simulink model "left_leg"  (R2014b)
settings: Solver=ode45  StartTime=0.0  StopTime=10  FixedStep=1e-4  RelTol=1e-3
undefined symbols (not defined in the file or in its folder): MX28_inertia, MX28_Te, X, Y, Z
libraries: sm_lib x39, nesl_utility x20
(part 1 of 2)
settings Model: Creator=florent  LastModifiedBy=florent
settings DebuggingCC: IntegerOverflowMsg=none  ParameterDowncastMsg=warning  ParameterPrecisionLossMsg=none  ParameterTunabilityLossMsg=none  StateNameClashWarn=warning  IntegerSaturationMsg=none

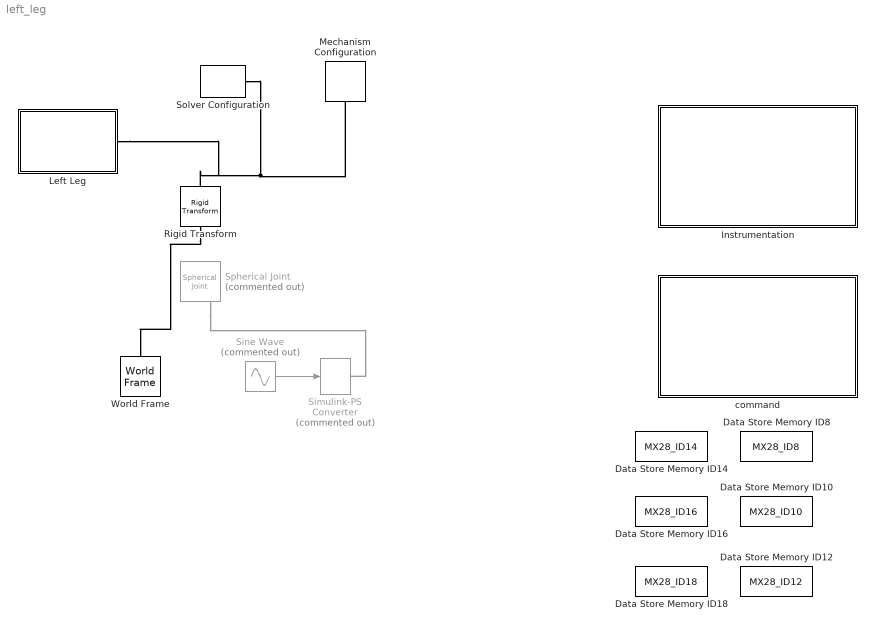
== system left_leg ==
  Data Store Memory ID10 : DataStoreMemory  DataStoreName=MX28_ID10  WriteAfterWriteMsg=error  InitialValue=MX28_default  VectorParams1D=off  OutDataTypeStr=Bus: MX28_bus
  Data Store Memory ID12 : DataStoreMemory  DataStoreName=MX28_ID12  WriteAfterWriteMsg=error  InitialValue=MX28_default  VectorParams1D=off  OutDataTypeStr=Bus: MX28_bus
  Data Store Memory ID14 : DataStoreMemory  DataStoreName=MX28_ID14  WriteAfterWriteMsg=error  InitialValue=MX28_default  VectorParams1D=off  OutDataTypeStr=Bus: MX28_bus
  Data Store Memory ID16 : DataStoreMemory  DataStoreName=MX28_ID16  WriteAfterWriteMsg=error  InitialValue=MX28_default  VectorParams1D=off  OutDataTypeStr=Bus: MX28_bus
  Data Store Memory ID18 : DataStoreMemory  DataStoreName=MX28_ID18  WriteAfterWriteMsg=error  InitialValue=MX28_default  VectorParams1D=off  OutDataTypeStr=Bus: MX28_bus
  Data Store Memory ID8 : DataStoreMemory  DataStoreName=MX28_ID8  WriteAfterWriteMsg=error  InitialValue=MX28_default  VectorParams1D=off  OutDataTypeStr=Bus: MX28_bus
  Instrumentation : Subsystem
  Left Leg : Subsystem
      mask init:
      | [ModelDir,~,~] = fileparts(which(gcs));
      | 
      | Block = [gcb '/Left Hip Yaw/Solid'];
      | STLFileName = [ModelDir filesep 'STL' filesep 'Hip1.STL'];
      | if ~strcmp(get_param(Block,'ExtGeomFileName'),STLFileName)
      |     set_param(Block,'ExtGeomFileName',STLFileName);
      | end
      | 
      | Block = [gcb '/Left Hip Roll/Solid'];
      | STLFileName = [ModelDir filesep 'STL' filesep 'Left_Hip2.STL'];
      | if ~strcmp(get_param(Block,'ExtGeomFileName'),STLFileName)
      |     set_param(Block,'ExtGeomFileName',STLFileName);
      | end
      | 
      | Block = [gcb '/Left Thigh/Solid'];
      | STLFileName = [ModelDir filesep 'STL' filesep 'Left_Thigh.STL'];
      | if ~strcmp(get_param(Block,'ExtGeomFileName'),STLFileName)
      |     set_param(Block,'ExtGeomFileName',STLFileName);
      | end
      | 
      | Block = [gcb '/Left Lower Leg/Solid'];
      | STLFileName = [ModelDir filesep 'STL' filesep 'Left_Lower_Leg.STL'];
      | if ~strcmp(get_param(Block,'ExtGeomFileName'),STLFileName)
      |     set_param(Block,'ExtGeomFileName',STLFileName);
      | end
      | 
      | Block = [gcb '/Left Ankle/Solid'];
      | STLFileName = [ModelDir filesep 'STL' filesep 'Left_Ankle.STL'];
      | if ~strcmp(get_param(Block,'ExtGeomFileName'),STLFileName)
      |     set_param(Block,'ExtGeomFileName',STLFileName);
      | end
      | 
      | Block = [gcb '/Left Foot/Solid'];
      | STLFileName = [ModelDir filesep 'STL' filesep 'Left_Foot.STL'];
      | if ~strcmp(get_param(Block,'ExtGeomFileName'),STLFileName)
      |     set_param(Block,'ExtGeomFileName',STLFileName);
      | end
  Mechanism Configuration : sm_lib/Utilities/Mechanism Configuration  UniformGravity=Constant  GravityVector=[0 0 -9.80665]  GravityUnits=m/s^2  LinearizationDelta=0.001  BlockFunction=simmechanics.library.utilities.mechanism_configuration
  Rigid Transform : sm_lib/Frames and Transforms/Rigid Transform  TranslationMethod=Cartesian  TranslationLengthUnit=m  TranslationStandardAxis=+Z  TranslationStandardOffset=0  TranslationCartesianOffset=[0 -0.001 0]  TranslationROffset=0  TranslationROffsetUnits=m  TranslationZOffset=0  TranslationZOffsetUnits=m  TranslationThetaOffset=0  TranslationThetaOffsetUnits=deg  RotationMethod=AlignedAxes  RotationAngleUnits=deg  RotationStandardAxis=+Z  RotationAngle=0  RotationArbitraryAxis=[0 0 1]  FollAlignAxisA=+Z  BaseAlignAxisA=-Z  FollAlignAxisB=+X  BaseAlignAxisB=-Y  RotationMatrix=[1 0 0; 0 1 0; 0 0 1]  BlockFunction=simmechanics.library.frames_transforms.rigid_transform
  Simulink-PS Converter : nesl_utility/Simulink-PS Converter  Commented=on  PhysicalDomain=network_engine_domain  SubClassName=ps_input  LeftPortType=input  RightPortType=output  PseudoPeriodic=off  Frequencies=[]  NoiseDistribution=none  NoiseParameters=[]  Unit=1  AffineConversion=off  InputFiltering=off  SimscapeFilterOrder=1  InputFilterTimeConstant=0.001  UdotUserProvided=1
  Sine Wave : Sin  Commented=on  Amplitude=0  Frequency=10  SampleTime=0
  Solver Configuration : nesl_utility/Solver Configuration  PhysicalDomain=network_engine_domain  SubClassName=solver  LeftPortType=input  RightPortType=generic  Accelerate=off  Tones=[]  Harmonics=[]  SimulateNoise=off  Profile=off  UseLocalSampling=off  EnableSwitchedLinearOptims=on  FrequencyDomain=off  UseCCode=off  RelTol=0.001  AbsTol=1e-06  MinStep=1e-09  ToWorkspace=off  DoDC=off  ResidualTolerance=1e-03  UseLocalSolver=on  LocalSolverChoice=NE_BACKWARD_EULER_ADVANCER  LocalSolverSampleTime=0.0001  DoFixedCost=on  MaxNonlinIter=3  MaxModeIter=2  LinearAlgebra=Sparse  DelaysMemoryBudget=1024  AutomaticFiltering=on  FilteringTimeConstant=0.001
  Spherical Joint : sm_lib/Joints/Spherical Joint  Commented=on  SenseConstraintForce=off  SenseConstraintForceX=off  SenseConstraintForceY=off  SenseConstraintForceZ=off  SenseConstraintTorque=off  SenseConstraintTorqueX=off  SenseConstraintTorqueY=off  SenseConstraintTorqueZ=off  SenseTotalForce=off  SenseTotalForceX=off  SenseTotalForceY=off  SenseTotalForceZ=off  SenseTotalTorque=off  SenseTotalTorqueX=off  SenseTotalTorqueY=off  SenseTotalTorqueZ=off  CompositeWrenchDir=FollowerOnBase  CompositeWrenchFrame=BaseFrame  DefPosRotationMethod=None  DefPosRotationAngleUnits=deg  DefPosRotationStandardAxis=+Z  DefPosRotationAngle=0  DefPosRotationArbitraryAxis=[0 0 1]  DefPosFollAlignAxisA=+X  DefPosBaseAlignAxisA=+Y  DefPosFollAlignAxisB=+Y  DefPosBaseAlignAxisB=+Z  DefPosRotationMatrix=[1 0 0; 0 1 0; 0 0 1]  EqPosRotationMethod=None  EqPosRotationAngleUnits=deg  EqPosRotationStandardAxis=+Z  EqPosRotationAngle=0  EqPosRotationArbitraryAxis=[0 0 1]  EqPosFollAlignAxisA=+X  EqPosBaseAlignAxisA=+Y  EqPosFollAlignAxisB=+Y  EqPosBaseAlignAxisB=+Z  EqPosRotationMatrix=[1 0 0; 0 1 0; 0 0 1]  SpringStiffness=0  SpringStiffnessUnits=N*m/deg  DampingCoefficient=0  DampingCoefficientUnits=N*m/(deg/s)  ActuateTorqueX=off  ActuateTorqueY=on  ActuateTorqueZ=off  ActuateTorque=off  TorqueActuationMode=InputTorque  MotionActuationMode=ComputedMotion  ActuationFrame=BaseFrame  SensePosition=off  SenseVelocityX=off  SenseVelocityY=off  SenseVelocityZ=off  SenseVelocity=off  SenseAccelerationX=off  SenseAccelerationY=off  SenseAccelerationZ=off  SenseAcceleration=off  SenseTorqueX=off  SenseTorqueY=off  SenseTorqueZ=off  SenseTorqueForce=off  SensingFrame=BaseFrame  PositionTargetRotationMethod=ArbitraryAxis  PositionTargetRotationAngleUnits=deg  PositionTargetRotationStandardAxis=+Z  PositionTargetRotationAngle=0  PositionTargetRotationArbitraryAxis=[0 -1 0]  PositionTargetFollAlignAxisA=+X  PositionTargetBaseAlignAxisA=+Y  PositionTargetFollAlignAxisB=+Y  PositionTargetBaseAlignAxisB=+Z  PositionTargetRotationMatrix=[1 0 0; 0 1 0; 0 0 1]  PositionTargetSpecify=on  PositionTargetPriority=High  VelocityTargetValue=[0 0 0]  VelocityTargetValueUnits=deg/s  VelocityTargetSpecify=off  VelocityTargetPriority=High  VelocityTargetInFollowerFrame=on  BlockFunction=simmechanics.library.joints.spherical_joint
  World Frame : sm_lib/Frames and Transforms/World Frame  BlockFunction=simmechanics.library.frames_transforms.world_frame
  command : Subsystem
  wires:
  Sine Wave/1 -> Simulink-PS Converter/1
  connections:
  Solver Configuration/RConn1 -- Left Leg/RConn1 -- Rigid Transform/RConn1 -- Mechanism Configuration/RConn1
  Rigid Transform/LConn1 -- World Frame/RConn1
  Spherical Joint/LConn2 -- Simulink-PS Converter/RConn1

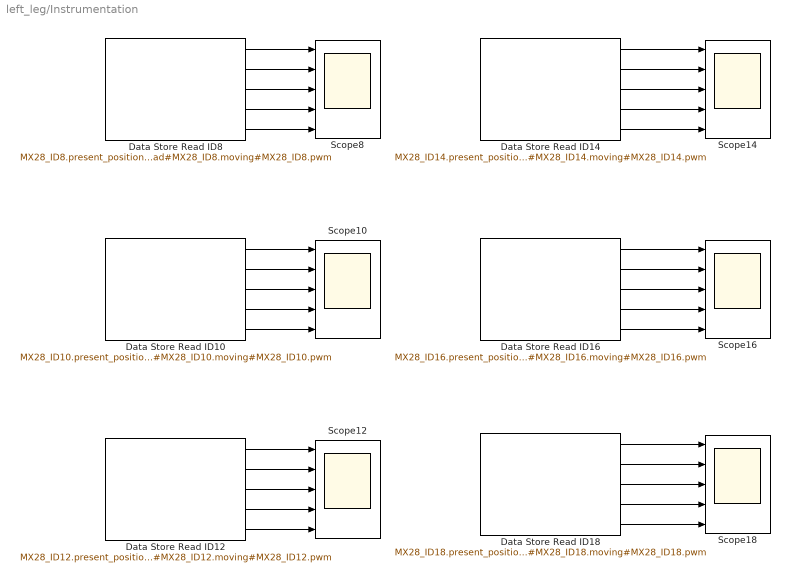
== system left_leg/Instrumentation ==
  Data Store Read ID10 : DataStoreRead  DataStoreName=MX28_ID10  SampleTime=0.001  DataStoreElements=MX28_ID10.present_position#MX28_ID10.present_speed#MX28_ID10.present_load#MX28_ID10.moving#MX28_ID10.pwm
  Data Store Read ID12 : DataStoreRead  DataStoreName=MX28_ID12  SampleTime=0.001  DataStoreElements=MX28_ID12.present_position#MX28_ID12.present_speed#MX28_ID12.present_load#MX28_ID12.moving#MX28_ID12.pwm
  Data Store Read ID14 : DataStoreRead  DataStoreName=MX28_ID14  SampleTime=0.001  DataStoreElements=MX28_ID14.present_position#MX28_ID14.present_speed#MX28_ID14.present_load#MX28_ID14.moving#MX28_ID14.pwm
  Data Store Read ID16 : DataStoreRead  DataStoreName=MX28_ID16  SampleTime=0.001  DataStoreElements=MX28_ID16.present_position#MX28_ID16.present_speed#MX28_ID16.present_load#MX28_ID16.moving#MX28_ID16.pwm
  Data Store Read ID18 : DataStoreRead  DataStoreName=MX28_ID18  SampleTime=0.001  DataStoreElements=MX28_ID18.present_position#MX28_ID18.present_speed#MX28_ID18.present_load#MX28_ID18.moving#MX28_ID18.pwm
  Data Store Read ID8 : DataStoreRead  DataStoreName=MX28_ID8  SampleTime=0.001  DataStoreElements=MX28_ID8.present_position#MX28_ID8.present_speed#MX28_ID8.present_load#MX28_ID8.moving#MX28_ID8.pwm
  Scope{8,10,12,14,16,18} (6 alike) : Scope  NumInputPorts=5
      Scope10 settings: YMin=-5~0~-5~-5~-5  YMax=5~650~5~5~5
      Scope12 settings: YMin=-5~0~-5~-5~-5  YMax=5~650~5~5~5
      Scope14 settings: YMin=-5~0~-5~-5~-5  YMax=5~650~5~5~5  SaveName=ScopeData3
      Scope16 settings: YMin=-5~0~-5~-5~-5  YMax=5~650~5~5~5  SaveName=ScopeData4
      Scope18 settings: YMin=-5~0~-5~-5~-5  YMax=5~650~5~5~5  SaveName=ScopeData5
      Scope8 settings: YMin=-5~0~-5~-5~-5  YMax=5~650~5~5~5  SaveName=ScopeData2
  wires:
  Data Store Read ID8/1 -> Scope8/1
  Data Store Read ID8/2 -> Scope8/2
  Data Store Read ID8/3 -> Scope8/3
  Data Store Read ID8/4 -> Scope8/4
  Data Store Read ID8/5 -> Scope8/5
  Data Store Read ID10/1 -> Scope10/1
  Data Store Read ID10/2 -> Scope10/2
  Data Store Read ID10/3 -> Scope10/3
  Data Store Read ID10/4 -> Scope10/4
  Data Store Read ID10/5 -> Scope10/5
  Data Store Read ID12/1 -> Scope12/1
  Data Store Read ID12/2 -> Scope12/2
  Data Store Read ID12/3 -> Scope12/3
  Data Store Read ID12/4 -> Scope12/4
  Data Store Read ID12/5 -> Scope12/5
  Data Store Read ID14/1 -> Scope14/1
  Data Store Read ID14/2 -> Scope14/2
  Data Store Read ID14/3 -> Scope14/3
  Data Store Read ID14/4 -> Scope14/4
  Data Store Read ID14/5 -> Scope14/5
  Data Store Read ID16/1 -> Scope16/1
  Data Store Read ID16/2 -> Scope16/2
  Data Store Read ID16/3 -> Scope16/3
  Data Store Read ID16/4 -> Scope16/4
  Data Store Read ID16/5 -> Scope16/5
  Data Store Read ID18/1 -> Scope18/1
  Data Store Read ID18/2 -> Scope18/2
  Data Store Read ID18/3 -> Scope18/3
  Data Store Read ID18/5 -> Scope18/5
  Data Store Read ID18/4 -> Scope18/4

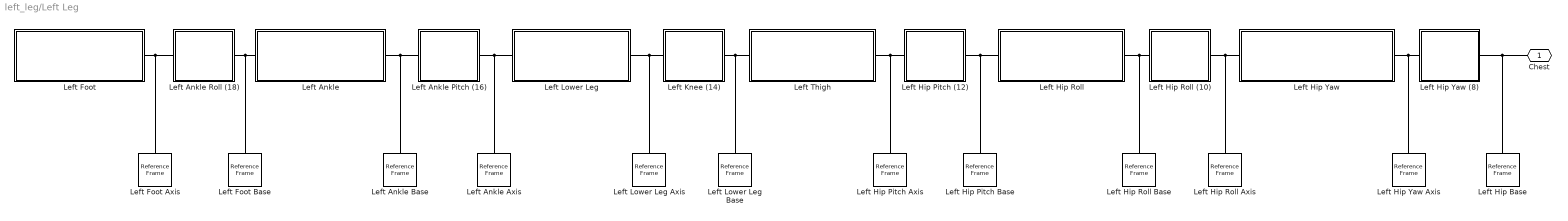
== system left_leg/Left Leg ==
  Left Ankle : Subsystem
  Left Ankle Axis : sm_lib/Frames and Transforms/Reference Frame  BlockFunction=simmechanics.library.frames_transforms.reference_frame
  Left Ankle Base : sm_lib/Frames and Transforms/Reference Frame  BlockFunction=simmechanics.library.frames_transforms.reference_frame
  Left Ankle Pitch (16) : Subsystem
  Left Ankle Roll (18) : Subsystem
  Left Foot : Subsystem
  Left Foot Axis : sm_lib/Frames and Transforms/Reference Frame  BlockFunction=simmechanics.library.frames_transforms.reference_frame
  Left Foot Base : sm_lib/Frames and Transforms/Reference Frame  BlockFunction=simmechanics.library.frames_transforms.reference_frame
  Left Hip Base : sm_lib/Frames and Transforms/Reference Frame  BlockFunction=simmechanics.library.frames_transforms.reference_frame
  Left Hip Pitch (12) : Subsystem
  Left Hip Pitch Axis : sm_lib/Frames and Transforms/Reference Frame  BlockFunction=simmechanics.library.frames_transforms.reference_frame
  Left Hip Pitch Base : sm_lib/Frames and Transforms/Reference Frame  BlockFunction=simmechanics.library.frames_transforms.reference_frame
  Left Hip Roll : Subsystem
  Left Hip Roll (10) : Subsystem
  Left Hip Roll Axis : sm_lib/Frames and Transforms/Reference Frame  BlockFunction=simmechanics.library.frames_transforms.reference_frame
  Left Hip Roll Base : sm_lib/Frames and Transforms/Reference Frame  BlockFunction=simmechanics.library.frames_transforms.reference_frame
  Left Hip Yaw : Subsystem
  Left Hip Yaw (8) : Subsystem
  Left Hip Yaw Axis : sm_lib/Frames and Transforms/Reference Frame  BlockFunction=simmechanics.library.frames_transforms.reference_frame
  Left Knee (14) : Subsystem
  Left Lower Leg : Subsystem
  Left Lower Leg Axis : sm_lib/Frames and Transforms/Reference Frame  BlockFunction=simmechanics.library.frames_transforms.reference_frame
  Left Lower Leg Base : sm_lib/Frames and Transforms/Reference Frame  BlockFunction=simmechanics.library.frames_transforms.reference_frame
  Left Thigh : Subsystem
  Chest : PMIOPort  Port=1  Side=Right
  connections:
  Chest/RConn1 -- Left Hip Yaw (8)/LConn1 -- Left Hip Base/RConn1
  Left Hip Roll/RConn1 -- Left Hip Pitch (12)/LConn1 -- Left Hip Pitch Base/RConn1
  Left Thigh/RConn1 -- Left Knee (14)/LConn1 -- Left Lower Leg Base/RConn1
  Left Lower Leg/RConn1 -- Left Ankle Pitch (16)/RConn1 -- Left Ankle Axis/RConn1
  Left Ankle/RConn1 -- Left Ankle Roll (18)/LConn1 -- Left Foot Base/RConn1
  Left Hip Yaw/LConn1 -- Left Hip Yaw (8)/RConn1 -- Left Hip Yaw Axis/RConn1
  Left Hip Roll Axis/RConn1 -- Left Hip Roll (10)/RConn1 -- Left Hip Yaw/RConn1
  Left Hip Roll Base/RConn1 -- Left Hip Roll (10)/LConn1 -- Left Hip Roll/LConn1
  Left Thigh/LConn1 -- Left Hip Pitch (12)/RConn1 -- Left Hip Pitch Axis/RConn1
  Left Lower Leg/LConn1 -- Left Knee (14)/RConn1 -- Left Lower Leg Axis/RConn1
  Left Ankle/LConn1 -- Left Ankle Pitch (16)/LConn1 -- Left Ankle Base/RConn1
  Left Foot/LConn1 -- Left Ankle Roll (18)/RConn1 -- Left Foot Axis/RConn1

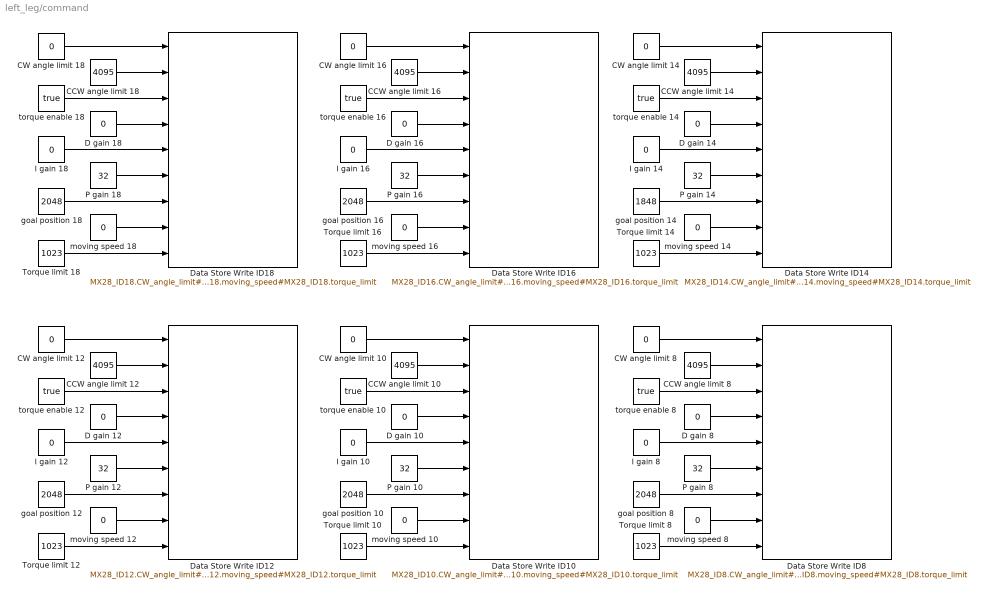
== system left_leg/command ==
  CCW angle limit {8,10,12,14,16,18} (6 alike) : Constant  Value=4095  OutDataTypeStr=int16
  CW angle limit {8,10,12,14,16,18} (6 alike) : Constant  Value=0  OutDataTypeStr=int16
  D gain {8,10,12,14,16,18} (6 alike) : Constant  Value=0  OutDataTypeStr=uint8
  Data Store Write ID10 : DataStoreWrite  DataStoreName=MX28_ID10  DataStoreElements=MX28_ID10.CW_angle_limit#MX28_ID10.CCW_angle_limit#MX28_ID10.torque_enable#MX28_ID10.D_gain#MX28_ID10.I_gain#MX28_ID10.P_gain#MX28_ID10.goal_position#MX28_ID10.moving_speed#MX28_ID10.torque_limit
  Data Store Write ID12 : DataStoreWrite  DataStoreName=MX28_ID12  DataStoreElements=MX28_ID12.CW_angle_limit#MX28_ID12.CCW_angle_limit#MX28_ID12.torque_enable#MX28_ID12.D_gain#MX28_ID12.I_gain#MX28_ID12.P_gain#MX28_ID12.goal_position#MX28_ID12.moving_speed#MX28_ID12.torque_limit
  Data Store Write ID14 : DataStoreWrite  DataStoreName=MX28_ID14  DataStoreElements=MX28_ID14.CW_angle_limit#MX28_ID14.CCW_angle_limit#MX28_ID14.torque_enable#MX28_ID14.D_gain#MX28_ID14.I_gain#MX28_ID14.P_gain#MX28_ID14.goal_position#MX28_ID14.moving_speed#MX28_ID14.torque_limit
  Data Store Write ID16 : DataStoreWrite  DataStoreName=MX28_ID16  DataStoreElements=MX28_ID16.CW_angle_limit#MX28_ID16.CCW_angle_limit#MX28_ID16.torque_enable#MX28_ID16.D_gain#MX28_ID16.I_gain#MX28_ID16.P_gain#MX28_ID16.goal_position#MX28_ID16.moving_speed#MX28_ID16.torque_limit
  Data Store Write ID18 : DataStoreWrite  DataStoreName=MX28_ID18  DataStoreElements=MX28_ID18.CW_angle_limit#MX28_ID18.CCW_angle_limit#MX28_ID18.torque_enable#MX28_ID18.D_gain#MX28_ID18.I_gain#MX28_ID18.P_gain#MX28_ID18.goal_position#MX28_ID18.moving_speed#MX28_ID18.torque_limit
  Data Store Write ID8 : DataStoreWrite  DataStoreName=MX28_ID8  DataStoreElements=MX28_ID8.CW_angle_limit#MX28_ID8.CCW_angle_limit#MX28_ID8.torque_enable#MX28_ID8.D_gain#MX28_ID8.I_gain#MX28_ID8.P_gain#MX28_ID8.goal_position#MX28_ID8.moving_speed#MX28_ID8.torque_limit
  I gain {8,10,12,14,16,18} (6 alike) : Constant  Value=0  OutDataTypeStr=uint8
  P gain {8,10,12,14,16,18} (6 alike) : Constant  Value=32  OutDataTypeStr=uint8
  Torque limit {8,10,12,14,16,18} (6 alike) : Constant  Value=1023  OutDataTypeStr=int16
  goal position {8,10,12,16,18} (5 alike) : Constant  Value=2048  OutDataTypeStr=int16
  goal position 14 : Constant  Value=1848  OutDataTypeStr=int16
  moving speed {8,10,12,14,16,18} (6 alike) : Constant  Value=0  OutDataTypeStr=int16
  torque enable {8,10,12,14,16,18} (6 alike) : Constant  Value=true  OutDataTypeStr=boolean
  wires:
  Torque limit 18/1 -> Data Store Write ID18/9
  moving speed 18/1 -> Data Store Write ID18/8
  goal position 18/1 -> Data Store Write ID18/7
  P gain 18/1 -> Data Store Write ID18/6
  I gain 18/1 -> Data Store Write ID18/5
  D gain 18/1 -> Data Store Write ID18/4
  torque enable 18/1 -> Data Store Write ID18/3
  CW angle limit 18/1 -> Data Store Write ID18/1
  CCW angle limit 18/1 -> Data Store Write ID18/2
  Torque limit 16/1 -> Data Store Write ID16/9
  moving speed 16/1 -> Data Store Write ID16/8
  goal position 16/1 -> Data Store Write ID16/7
  P gain 16/1 -> Data Store Write ID16/6
  I gain 16/1 -> Data Store Write ID16/5
  D gain 16/1 -> Data Store Write ID16/4
  torque enable 16/1 -> Data Store Write ID16/3
  CCW angle limit 16/1 -> Data Store Write ID16/2
  CW angle limit 16/1 -> Data Store Write ID16/1
  Torque limit 14/1 -> Data Store Write ID14/9
  moving speed 14/1 -> Data Store Write ID14/8
  goal position 14/1 -> Data Store Write ID14/7
  P gain 14/1 -> Data Store Write ID14/6
  I gain 14/1 -> Data Store Write ID14/5
  D gain 14/1 -> Data Store Write ID14/4
  torque enable 14/1 -> Data Store Write ID14/3
  CW angle limit 14/1 -> Data Store Write ID14/1
  CCW angle limit 14/1 -> Data Store Write ID14/2
  Torque limit 12/1 -> Data Store Write ID12/9
  moving speed 12/1 -> Data Store Write ID12/8
  goal position 12/1 -> Data Store Write ID12/7
  P gain 12/1 -> Data Store Write ID12/6
  I gain 12/1 -> Data Store Write ID12/5
  D gain 12/1 -> Data Store Write ID12/4
  torque enable 12/1 -> Data Store Write ID12/3
  CCW angle limit 12/1 -> Data Store Write ID12/2
  CW angle limit 12/1 -> Data Store Write ID12/1
  Torque limit 10/1 -> Data Store Write ID10/9
  moving speed 10/1 -> Data Store Write ID10/8
  goal position 10/1 -> Data Store Write ID10/7
  P gain 10/1 -> Data Store Write ID10/6
  I gain 10/1 -> Data Store Write ID10/5
  D gain 10/1 -> Data Store Write ID10/4
  torque enable 10/1 -> Data Store Write ID10/3
  CW angle limit 10/1 -> Data Store Write ID10/1
  CCW angle limit 10/1 -> Data Store Write ID10/2
  Torque limit 8/1 -> Data Store Write ID8/9
  moving speed 8/1 -> Data Store Write ID8/8
  goal position 8/1 -> Data Store Write ID8/7
  P gain 8/1 -> Data Store Write ID8/6
  I gain 8/1 -> Data Store Write ID8/5
  D gain 8/1 -> Data Store Write ID8/4
  torque enable 8/1 -> Data Store Write ID8/3
  CW angle limit 8/1 -> Data Store Write ID8/1
  CCW angle limit 8/1 -> Data Store Write ID8/2

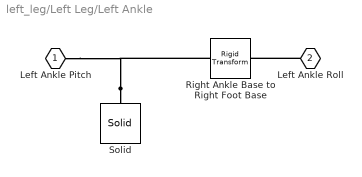
== system left_leg/Left Leg/Left Ankle ==
  Right Ankle Base to Right Foot Base : sm_lib/Frames and Transforms/Rigid Transform  TranslationMethod=Cartesian  TranslationLengthUnit=mm  TranslationStandardAxis=+Z  TranslationStandardOffset=0  TranslationCartesianOffset=[19.35 0 -23.55]  TranslationROffset=0  TranslationROffsetUnits=m  TranslationZOffset=0  TranslationZOffsetUnits=m  TranslationThetaOffset=0  TranslationThetaOffsetUnits=deg  RotationMethod=AlignedAxes  RotationAngleUnits=deg  RotationStandardAxis=+Z  RotationAngle=0  RotationArbitraryAxis=[0 0 1]  FollAlignAxisA=+X  BaseAlignAxisA=-Z  FollAlignAxisB=+Y  BaseAlignAxisB=-Y  RotationMatrix=[1 0 0; 0 1 0; 0 0 1]  BlockFunction=simmechanics.library.frames_transforms.rigid_transform
  Solid : sm_lib/Body Elements/Solid  InertiaType=Custom  Mass=166.79  MassUnits=g  CenterOfMass=[18.06 -11.21 -23.86]  CenterOfMassUnits=mm  MomentsOfInertia=[6949 12213 11817]  MomentsOfInertiaUnits=g*mm^2  ProductsOfInertia=[-199 -104 -4006]  ProductsOfInertiaUnits=g*mm^2  DensityBased=on  Density=1000  DensityUnits=kg/(m^3)  GraphicType=FromGeometry  MarkerShape=Sphere  MarkerSize=10  MarkerSizeUnits=m  GraphicVisPropType=SimpleVisualProperties  GraphicDiffuseColor=[0.5 0.5 0.5]  GraphicSpecularColor=[0.5 0.5 0.5 1.0]  GraphicAmbientColor=[0.15 0.15 0.15 1.0]  GraphicEmissiveColor=[0.0 0.0 0.0 1.0]  GraphicShininess=75  GraphicOpacity=1.0  GeometryShape=FromFile  RectangleSize=[1 1]  RectangleSizeUnits=m  BrickDimensions=[1 1 1]  BrickDimensionUnits=m  CylinderRadius=1  CylinderRadiusUnits=m  CylinderLength=1  CylinderLengthUnits=m  SphereRadius=1  SphereRadiusUnits=m  EllipsoidRadii=[1 1 1]  EllipsoidRadiiUnits=m  ExtrusionCrossSection=[1 1; -1 1; -1 -1; 1 -1]  ExtrusionCrossSectionUnits=m  ExtrusionLength=1  ExtrusionLengthUnits=m  PolygonNumSides=3  PolygonOuterRadius=1  PolygonOuterRadiusUnits=m  ExtGeomFileType=STL  ExtGeomFileName=D:\Ker Lann\systemes\darwin\kinematics\STL\Left_Ankle.STL  ExtGeomFileUnits=mm  RevolutionCrossSection=[1 1; 1 -1; 2 -1; 2 1]  RevolutionCrossSectionUnits=m  RevolutionExtent=Full  RevolutionAngle=180  RevolutionAngleUnits=deg  BlockFunction=simmechanics.library.body_elements.solid
  Left Ankle Pitch : PMIOPort  Port=1  Side=Left
  Left Ankle Roll : PMIOPort  Port=2  Side=Right
  connections:
  Solid/RConn1 -- Right Ankle Base to Right Foot Base/LConn1 -- Left Ankle Pitch/RConn1
  Left Ankle Roll/RConn1 -- Right Ankle Base to Right Foot Base/RConn1

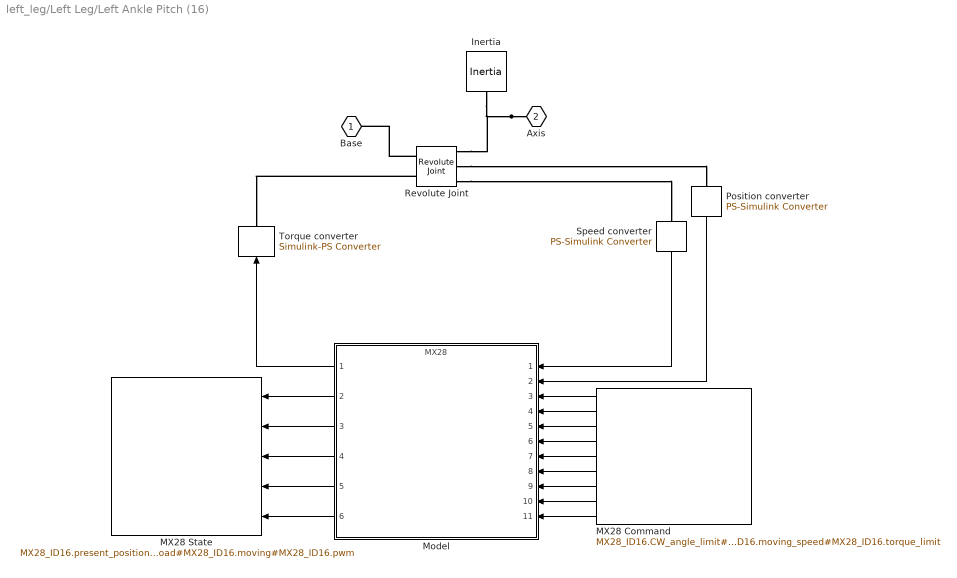
== system left_leg/Left Leg/Left Ankle Pitch (16) ==
  Inertia : sm_lib/Body Elements/Inertia  InertiaType=Custom  Mass=1  MassUnits=g  CenterOfMass=[0 0 0]  CenterOfMassUnits=m  MomentsOfInertia=[0 0 MX28_inertia]  MomentsOfInertiaUnits=kg*m^2  ProductsOfInertia=[0 0 0]  ProductsOfInertiaUnits=kg*m^2  BlockFunction=simmechanics.library.body_elements.inertia
  MX28 Command : DataStoreRead  DataStoreName=MX28_ID16  SampleTime=MX28_Te  DataStoreElements=MX28_ID16.CW_angle_limit#MX28_ID16.CCW_angle_limit#MX28_ID16.torque_enable#MX28_ID16.D_gain#MX28_ID16.I_gain#MX28_ID16.P_gain#MX28_ID16.goal_position#MX28_ID16.moving_speed#MX28_ID16.torque_limit
  MX28 State : DataStoreWrite  DataStoreName=MX28_ID16  DataStoreElements=MX28_ID16.present_position#MX28_ID16.present_speed#MX28_ID16.present_load#MX28_ID16.moving#MX28_ID16.pwm
  Model : ModelReference  ModelNameDialog=MX28.slx  SimulationMode=Normal  ModelReferenceVersion=1.66  CopyOfModelName=MX28.slx  DefaultDataLogging=on
  Position converter : nesl_utility/PS-Simulink Converter  PhysicalDomain=network_engine_domain  SubClassName=ps_output  LeftPortType=input  RightPortType=output  PseudoPeriodic=off  Frequencies=[]  Unit=rad  AffineConversion=off
  Revolute Joint : sm_lib/Joints/Revolute Joint  SenseConstraintForce=off  SenseConstraintForceX=off  SenseConstraintForceY=off  SenseConstraintForceZ=off  SenseConstraintTorque=off  SenseConstraintTorqueX=off  SenseConstraintTorqueY=off  SenseConstraintTorqueZ=off  SenseTotalForce=off  SenseTotalForceX=off  SenseTotalForceY=off  SenseTotalForceZ=off  SenseTotalTorque=off  SenseTotalTorqueX=off  SenseTotalTorqueY=off  SenseTotalTorqueZ=off  CompositeWrenchDir=FollowerOnBase  CompositeWrenchFrame=BaseFrame  EquilibriumPosition=0  EquilibriumPositionUnits=deg  SpringStiffness=0  SpringStiffnessUnits=N*m/deg  DampingCoefficient=MX28_lub_friction  DampingCoefficientUnits=N*m/(rad/s)  TorqueActuationMode=InputTorque  MotionActuationMode=ComputedMotion  SensePosition=on  SenseVelocity=on  SenseAcceleration=off  SenseTorqueForce=off  PositionTargetValue=MX28_init_position  PositionTargetValueUnits=rad  PositionTargetSpecify=on  PositionTargetPriority=High  VelocityTargetValue=MX28_init_speed  VelocityTargetValueUnits=rad/s  VelocityTargetSpecify=on  VelocityTargetPriority=High  BlockFunction=simmechanics.library.joints.revolute_joint
  Speed converter : nesl_utility/PS-Simulink Converter  PhysicalDomain=network_engine_domain  SubClassName=ps_output  LeftPortType=input  RightPortType=output  PseudoPeriodic=off  Frequencies=[]  Unit=rad/s  AffineConversion=off
  Torque converter : nesl_utility/Simulink-PS Converter  PhysicalDomain=network_engine_domain  SubClassName=ps_input  LeftPortType=input  RightPortType=output  PseudoPeriodic=off  Frequencies=[]  NoiseDistribution=none  NoiseParameters=[]  Unit=N*m  AffineConversion=off  InputFiltering=off  SimscapeFilterOrder=1  InputFilterTimeConstant=0.001  UdotUserProvided=1
  Base : PMIOPort  Port=1  Side=Left
  Axis : PMIOPort  Port=2  Side=Right
  wires:
  Model/4 -> MX28 State/3
  Model/2 -> MX28 State/1
  Model/5 -> MX28 State/4
  Model/3 -> MX28 State/2
  MX28 Command/3 -> Model/5
  MX28 Command/6 -> Model/8
  MX28 Command/4 -> Model/6
  MX28 Command/5 -> Model/7
  MX28 Command/7 -> Model/9
  MX28 Command/2 -> Model/4
  MX28 Command/1 -> Model/3
  Speed converter/1 -> Model/1
  Position converter/1 -> Model/2
  Model/1 -> Torque converter/1
  Model/6 -> MX28 State/5
  MX28 Command/8 -> Model/10
  MX28 Command/9 -> Model/11
  connections:
  Axis/RConn1 -- Revolute Joint/RConn1 -- Inertia/RConn1
  Revolute Joint/LConn1 -- Base/RConn1
  Revolute Joint/RConn3 -- Speed converter/LConn1
  Revolute Joint/RConn2 -- Position converter/LConn1
  Revolute Joint/LConn2 -- Torque converter/RConn1

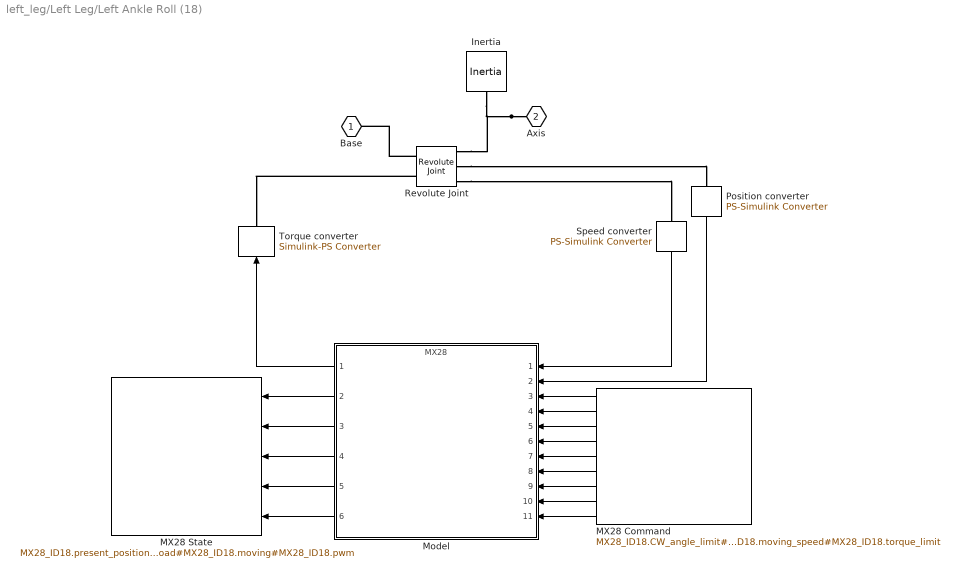
== system left_leg/Left Leg/Left Ankle Roll (18) ==
  Inertia : sm_lib/Body Elements/Inertia  InertiaType=Custom  Mass=1  MassUnits=g  CenterOfMass=[0 0 0]  CenterOfMassUnits=m  MomentsOfInertia=[0 0 MX28_inertia]  MomentsOfInertiaUnits=kg*m^2  ProductsOfInertia=[0 0 0]  ProductsOfInertiaUnits=kg*m^2  BlockFunction=simmechanics.library.body_elements.inertia
  MX28 Command : DataStoreRead  DataStoreName=MX28_ID18  SampleTime=MX28_Te  DataStoreElements=MX28_ID18.CW_angle_limit#MX28_ID18.CCW_angle_limit#MX28_ID18.torque_enable#MX28_ID18.D_gain#MX28_ID18.I_gain#MX28_ID18.P_gain#MX28_ID18.goal_position#MX28_ID18.moving_speed#MX28_ID18.torque_limit
  MX28 State : DataStoreWrite  DataStoreName=MX28_ID18  DataStoreElements=MX28_ID18.present_position#MX28_ID18.present_speed#MX28_ID18.present_load#MX28_ID18.moving#MX28_ID18.pwm
  Model : ModelReference  ModelNameDialog=MX28.slx  SimulationMode=Normal  ModelReferenceVersion=1.66  CopyOfModelName=MX28.slx  DefaultDataLogging=on
  Position converter : nesl_utility/PS-Simulink Converter  PhysicalDomain=network_engine_domain  SubClassName=ps_output  LeftPortType=input  RightPortType=output  PseudoPeriodic=off  Frequencies=[]  Unit=rad  AffineConversion=off
  Revolute Joint : sm_lib/Joints/Revolute Joint  SenseConstraintForce=off  SenseConstraintForceX=off  SenseConstraintForceY=off  SenseConstraintForceZ=off  SenseConstraintTorque=off  SenseConstraintTorqueX=off  SenseConstraintTorqueY=off  SenseConstraintTorqueZ=off  SenseTotalForce=off  SenseTotalForceX=off  SenseTotalForceY=off  SenseTotalForceZ=off  SenseTotalTorque=off  SenseTotalTorqueX=off  SenseTotalTorqueY=off  SenseTotalTorqueZ=off  CompositeWrenchDir=FollowerOnBase  CompositeWrenchFrame=BaseFrame  EquilibriumPosition=0  EquilibriumPositionUnits=deg  SpringStiffness=0  SpringStiffnessUnits=N*m/deg  DampingCoefficient=MX28_lub_friction  DampingCoefficientUnits=N*m/(rad/s)  TorqueActuationMode=InputTorque  MotionActuationMode=ComputedMotion  SensePosition=on  SenseVelocity=on  SenseAcceleration=off  SenseTorqueForce=off  PositionTargetValue=MX28_init_position  PositionTargetValueUnits=rad  PositionTargetSpecify=on  PositionTargetPriority=High  VelocityTargetValue=MX28_init_speed  VelocityTargetValueUnits=rad/s  VelocityTargetSpecify=on  VelocityTargetPriority=High  BlockFunction=simmechanics.library.joints.revolute_joint
  Speed converter : nesl_utility/PS-Simulink Converter  PhysicalDomain=network_engine_domain  SubClassName=ps_output  LeftPortType=input  RightPortType=output  PseudoPeriodic=off  Frequencies=[]  Unit=rad/s  AffineConversion=off
  Torque converter : nesl_utility/Simulink-PS Converter  PhysicalDomain=network_engine_domain  SubClassName=ps_input  LeftPortType=input  RightPortType=output  PseudoPeriodic=off  Frequencies=[]  NoiseDistribution=none  NoiseParameters=[]  Unit=N*m  AffineConversion=off  InputFiltering=off  SimscapeFilterOrder=1  InputFilterTimeConstant=0.001  UdotUserProvided=1
  Base : PMIOPort  Port=1  Side=Left
  Axis : PMIOPort  Port=2  Side=Right
  wires:
  Model/4 -> MX28 State/3
  Model/2 -> MX28 State/1
  Model/5 -> MX28 State/4
  Model/3 -> MX28 State/2
  MX28 Command/3 -> Model/5
  MX28 Command/6 -> Model/8
  MX28 Command/4 -> Model/6
  MX28 Command/5 -> Model/7
  MX28 Command/7 -> Model/9
  MX28 Command/2 -> Model/4
  MX28 Command/1 -> Model/3
  Speed converter/1 -> Model/1
  Position converter/1 -> Model/2
  Model/1 -> Torque converter/1
  Model/6 -> MX28 State/5
  MX28 Command/8 -> Model/10
  MX28 Command/9 -> Model/11
  connections:
  Axis/RConn1 -- Revolute Joint/RConn1 -- Inertia/RConn1
  Revolute Joint/LConn1 -- Base/RConn1
  Revolute Joint/RConn3 -- Speed converter/LConn1
  Revolute Joint/RConn2 -- Position converter/LConn1
  Revolute Joint/LConn2 -- Torque converter/RConn1

== system left_leg/Left Leg/Left Foot ==
  Solid : sm_lib/Body Elements/Solid  InertiaType=Custom  Mass=76.78  MassUnits=g  CenterOfMass=[-7.76 24.5 17.25]  CenterOfMassUnits=mm  MomentsOfInertia=[69069 85304 36676]  MomentsOfInertiaUnits=g*mm^2  ProductsOfInertia=[4062 -778 -2754]  ProductsOfInertiaUnits=g*mm^2  DensityBased=on  Density=1000  DensityUnits=kg/(m^3)  GraphicType=FromGeometry  MarkerShape=Sphere  MarkerSize=10  MarkerSizeUnits=m  GraphicVisPropType=SimpleVisualProperties  GraphicDiffuseColor=[0.5 0.5 0.5]  GraphicSpecularColor=[0.5 0.5 0.5 1.0]  GraphicAmbientColor=[0.15 0.15 0.15 1.0]  GraphicEmissiveColor=[0.0 0.0 0.0 1.0]  GraphicShininess=75  GraphicOpacity=1.0  GeometryShape=FromFile  RectangleSize=[1 1]  RectangleSizeUnits=m  BrickDimensions=[1 1 1]  BrickDimensionUnits=m  CylinderRadius=1  CylinderRadiusUnits=m  CylinderLength=1  CylinderLengthUnits=m  SphereRadius=1  SphereRadiusUnits=m  EllipsoidRadii=[1 1 1]  EllipsoidRadiiUnits=m  ExtrusionCrossSection=[1 1; -1 1; -1 -1; 1 -1]  ExtrusionCrossSectionUnits=m  ExtrusionLength=1  ExtrusionLengthUnits=m  PolygonNumSides=3  PolygonOuterRadius=1  PolygonOuterRadiusUnits=m  ExtGeomFileType=STL  ExtGeomFileName=D:\Ker Lann\systemes\darwin\kinematics\STL\Left_Foot.STL  ExtGeomFileUnits=mm  RevolutionCrossSection=[1 1; 1 -1; 2 -1; 2 1]  RevolutionCrossSectionUnits=m  RevolutionExtent=Full  RevolutionAngle=180  RevolutionAngleUnits=deg  BlockFunction=simmechanics.library.body_elements.solid
  Left Ankle Roll : PMIOPort  Port=1  Side=Left
  connections:
  Left Ankle Roll/RConn1 -- Solid/RConn1

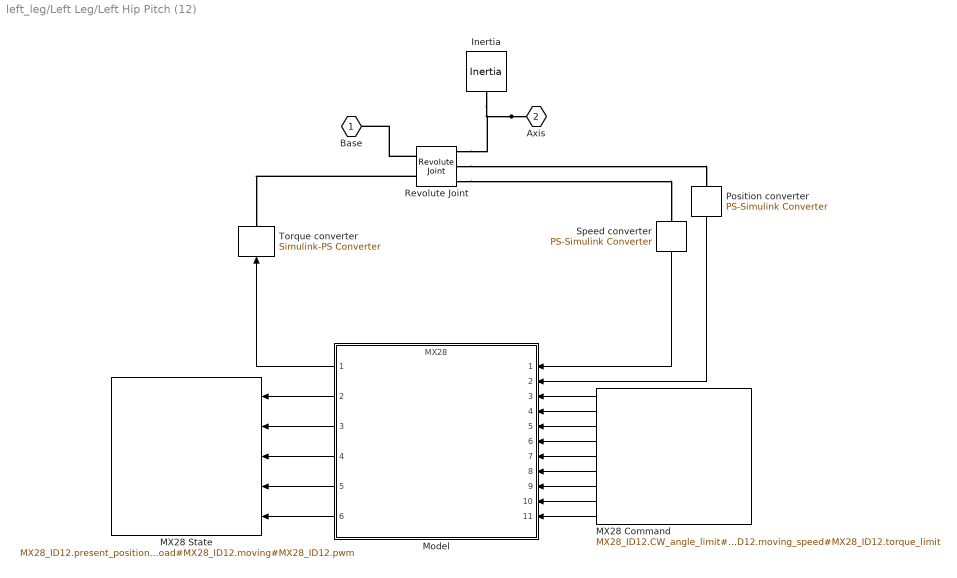
== system left_leg/Left Leg/Left Hip Pitch (12) ==
  Inertia : sm_lib/Body Elements/Inertia  InertiaType=Custom  Mass=1  MassUnits=g  CenterOfMass=[0 0 0]  CenterOfMassUnits=m  MomentsOfInertia=[0 0 MX28_inertia]  MomentsOfInertiaUnits=kg*m^2  ProductsOfInertia=[0 0 0]  ProductsOfInertiaUnits=kg*m^2  BlockFunction=simmechanics.library.body_elements.inertia
  MX28 Command : DataStoreRead  DataStoreName=MX28_ID12  SampleTime=MX28_Te  DataStoreElements=MX28_ID12.CW_angle_limit#MX28_ID12.CCW_angle_limit#MX28_ID12.torque_enable#MX28_ID12.D_gain#MX28_ID12.I_gain#MX28_ID12.P_gain#MX28_ID12.goal_position#MX28_ID12.moving_speed#MX28_ID12.torque_limit
  MX28 State : DataStoreWrite  DataStoreName=MX28_ID12  DataStoreElements=MX28_ID12.present_position#MX28_ID12.present_speed#MX28_ID12.present_load#MX28_ID12.moving#MX28_ID12.pwm
  Model : ModelReference  ModelNameDialog=MX28.slx  SimulationMode=Normal  ModelReferenceVersion=1.66  CopyOfModelName=MX28.slx  DefaultDataLogging=on
  Position converter : nesl_utility/PS-Simulink Converter  PhysicalDomain=network_engine_domain  SubClassName=ps_output  LeftPortType=input  RightPortType=output  PseudoPeriodic=off  Frequencies=[]  Unit=rad  AffineConversion=off
  Revolute Joint : sm_lib/Joints/Revolute Joint  SenseConstraintForce=off  SenseConstraintForceX=off  SenseConstraintForceY=off  SenseConstraintForceZ=off  SenseConstraintTorque=off  SenseConstraintTorqueX=off  SenseConstraintTorqueY=off  SenseConstraintTorqueZ=off  SenseTotalForce=off  SenseTotalForceX=off  SenseTotalForceY=off  SenseTotalForceZ=off  SenseTotalTorque=off  SenseTotalTorqueX=off  SenseTotalTorqueY=off  SenseTotalTorqueZ=off  CompositeWrenchDir=FollowerOnBase  CompositeWrenchFrame=BaseFrame  EquilibriumPosition=0  EquilibriumPositionUnits=deg  SpringStiffness=0  SpringStiffnessUnits=N*m/deg  DampingCoefficient=MX28_lub_friction  DampingCoefficientUnits=N*m/(rad/s)  TorqueActuationMode=InputTorque  MotionActuationMode=ComputedMotion  SensePosition=on  SenseVelocity=on  SenseAcceleration=off  SenseTorqueForce=off  PositionTargetValue=MX28_init_position  PositionTargetValueUnits=rad  PositionTargetSpecify=on  PositionTargetPriority=High  VelocityTargetValue=MX28_init_speed  VelocityTargetValueUnits=rad/s  VelocityTargetSpecify=on  VelocityTargetPriority=High  BlockFunction=simmechanics.library.joints.revolute_joint
  Speed converter : nesl_utility/PS-Simulink Converter  PhysicalDomain=network_engine_domain  SubClassName=ps_output  LeftPortType=input  RightPortType=output  PseudoPeriodic=off  Frequencies=[]  Unit=rad/s  AffineConversion=off
  Torque converter : nesl_utility/Simulink-PS Converter  PhysicalDomain=network_engine_domain  SubClassName=ps_input  LeftPortType=input  RightPortType=output  PseudoPeriodic=off  Frequencies=[]  NoiseDistribution=none  NoiseParameters=[]  Unit=N*m  AffineConversion=off  InputFiltering=off  SimscapeFilterOrder=1  InputFilterTimeConstant=0.001  UdotUserProvided=1
  Base : PMIOPort  Port=1  Side=Left
  Axis : PMIOPort  Port=2  Side=Right
  wires:
  Model/4 -> MX28 State/3
  Model/2 -> MX28 State/1
  Model/5 -> MX28 State/4
  Model/3 -> MX28 State/2
  MX28 Command/3 -> Model/5
  MX28 Command/6 -> Model/8
  MX28 Command/4 -> Model/6
  MX28 Command/5 -> Model/7
  MX28 Command/7 -> Model/9
  MX28 Command/2 -> Model/4
  MX28 Command/1 -> Model/3
  Speed converter/1 -> Model/1
  Position converter/1 -> Model/2
  Model/1 -> Torque converter/1
  Model/6 -> MX28 State/5
  MX28 Command/8 -> Model/10
  MX28 Command/9 -> Model/11
  connections:
  Axis/RConn1 -- Revolute Joint/RConn1 -- Inertia/RConn1
  Revolute Joint/LConn1 -- Base/RConn1
  Revolute Joint/RConn3 -- Speed converter/LConn1
  Revolute Joint/RConn2 -- Position converter/LConn1
  Revolute Joint/LConn2 -- Torque converter/RConn1

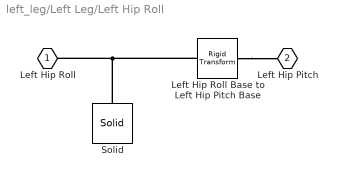
== system left_leg/Left Leg/Left Hip Roll ==
  Left Hip Roll Base to Left Hip Pitch Base : sm_lib/Frames and Transforms/Rigid Transform  TranslationMethod=Cartesian  TranslationLengthUnit=mm  TranslationStandardAxis=+Z  TranslationStandardOffset=0  TranslationCartesianOffset=[-23.9 0 19.1]  TranslationROffset=0  TranslationROffsetUnits=m  TranslationZOffset=0  TranslationZOffsetUnits=m  TranslationThetaOffset=0  TranslationThetaOffsetUnits=deg  RotationMethod=AlignedAxes  RotationAngleUnits=deg  RotationStandardAxis=+Z  RotationAngle=0  RotationArbitraryAxis=[0 0 1]  FollAlignAxisA=+Y  BaseAlignAxisA=+Y  FollAlignAxisB=+X  BaseAlignAxisB=+Z  RotationMatrix=[1 0 0; 0 1 0; 0 0 1]  BlockFunction=simmechanics.library.frames_transforms.rigid_transform
  Solid : sm_lib/Body Elements/Solid  InertiaType=Custom  Mass=166.79  MassUnits=g  CenterOfMass=[0.3 -11.21 1.04]  CenterOfMassUnits=mm  MomentsOfInertia=[11815 12217 6971]  MomentsOfInertiaUnits=g*mm^2  ProductsOfInertia=[4000 -134 178]  ProductsOfInertiaUnits=g*mm^2  DensityBased=on  Density=1000  DensityUnits=kg/(m^3)  GraphicType=FromGeometry  MarkerShape=Sphere  MarkerSize=10  MarkerSizeUnits=m  GraphicVisPropType=SimpleVisualProperties  GraphicDiffuseColor=[0.5 0.5 0.5]  GraphicSpecularColor=[0.5 0.5 0.5 1.0]  GraphicAmbientColor=[0.15 0.15 0.15 1.0]  GraphicEmissiveColor=[0.0 0.0 0.0 1.0]  GraphicShininess=75  GraphicOpacity=1.0  GeometryShape=FromFile  RectangleSize=[1 1]  RectangleSizeUnits=m  BrickDimensions=[1 1 1]  BrickDimensionUnits=mm  CylinderRadius=1  CylinderRadiusUnits=m  CylinderLength=1  CylinderLengthUnits=m  SphereRadius=1  SphereRadiusUnits=m  EllipsoidRadii=[1 1 1]  EllipsoidRadiiUnits=m  ExtrusionCrossSection=[1 1; -1 1; -1 -1; 1 -1]  ExtrusionCrossSectionUnits=m  ExtrusionLength=1  ExtrusionLengthUnits=m  PolygonNumSides=3  PolygonOuterRadius=1  PolygonOuterRadiusUnits=m  ExtGeomFileType=STL  ExtGeomFileName=D:\Ker Lann\systemes\darwin\kinematics\STL\Left_Hip2.STL  ExtGeomFileUnits=mm  RevolutionCrossSection=[1 1; 1 -1; 2 -1; 2 1]  RevolutionCrossSectionUnits=m  RevolutionExtent=Full  RevolutionAngle=180  RevolutionAngleUnits=deg  BlockFunction=simmechanics.library.body_elements.solid
  Left Hip Roll : PMIOPort  Port=1  Side=Left
  Left Hip Pitch : PMIOPort  Port=2  Side=Right
  connections:
  Left Hip Roll Base to Left Hip Pitch Base/LConn1 -- Solid/RConn1 -- Left Hip Roll/RConn1
  Left Hip Roll Base to Left Hip Pitch Base/RConn1 -- Left Hip Pitch/RConn1

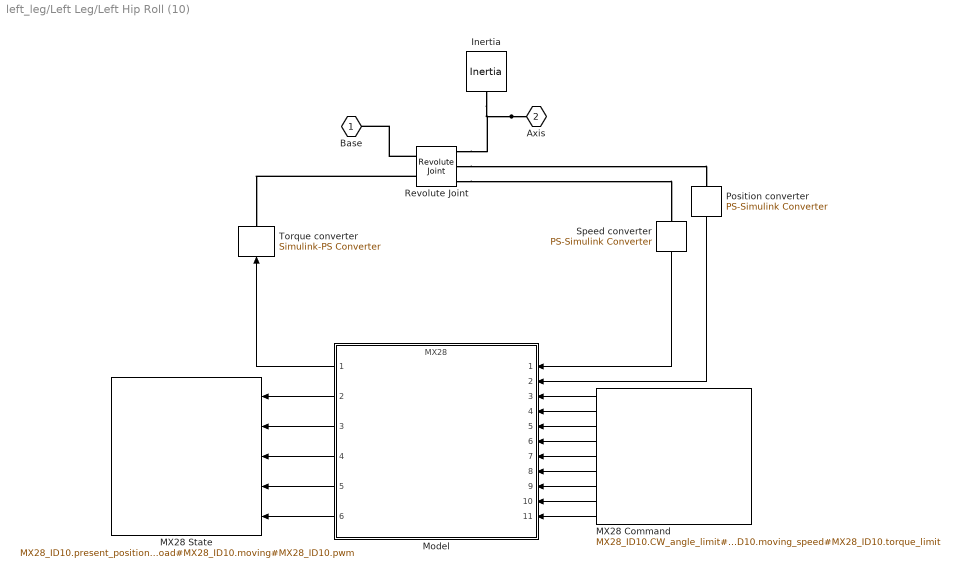
== system left_leg/Left Leg/Left Hip Roll (10) ==
  Inertia : sm_lib/Body Elements/Inertia  InertiaType=Custom  Mass=1  MassUnits=g  CenterOfMass=[0 0 0]  CenterOfMassUnits=m  MomentsOfInertia=[0 0 MX28_inertia]  MomentsOfInertiaUnits=kg*m^2  ProductsOfInertia=[0 0 0]  ProductsOfInertiaUnits=kg*m^2  BlockFunction=simmechanics.library.body_elements.inertia
  MX28 Command : DataStoreRead  DataStoreName=MX28_ID10  SampleTime=MX28_Te  DataStoreElements=MX28_ID10.CW_angle_limit#MX28_ID10.CCW_angle_limit#MX28_ID10.torque_enable#MX28_ID10.D_gain#MX28_ID10.I_gain#MX28_ID10.P_gain#MX28_ID10.goal_position#MX28_ID10.moving_speed#MX28_ID10.torque_limit
  MX28 State : DataStoreWrite  DataStoreName=MX28_ID10  DataStoreElements=MX28_ID10.present_position#MX28_ID10.present_speed#MX28_ID10.present_load#MX28_ID10.moving#MX28_ID10.pwm
  Model : ModelReference  ModelNameDialog=MX28.slx  SimulationMode=Normal  ModelReferenceVersion=1.66  CopyOfModelName=MX28.slx  DefaultDataLogging=on
  Position converter : nesl_utility/PS-Simulink Converter  PhysicalDomain=network_engine_domain  SubClassName=ps_output  LeftPortType=input  RightPortType=output  PseudoPeriodic=off  Frequencies=[]  Unit=rad  AffineConversion=off
  Revolute Joint : sm_lib/Joints/Revolute Joint  SenseConstraintForce=off  SenseConstraintForceX=off  SenseConstraintForceY=off  SenseConstraintForceZ=off  SenseConstraintTorque=off  SenseConstraintTorqueX=off  SenseConstraintTorqueY=off  SenseConstraintTorqueZ=off  SenseTotalForce=off  SenseTotalForceX=off  SenseTotalForceY=off  SenseTotalForceZ=off  SenseTotalTorque=off  SenseTotalTorqueX=off  SenseTotalTorqueY=off  SenseTotalTorqueZ=off  CompositeWrenchDir=FollowerOnBase  CompositeWrenchFrame=BaseFrame  EquilibriumPosition=0  EquilibriumPositionUnits=deg  SpringStiffness=0  SpringStiffnessUnits=N*m/deg  DampingCoefficient=MX28_lub_friction  DampingCoefficientUnits=N*m/(rad/s)  TorqueActuationMode=InputTorque  MotionActuationMode=ComputedMotion  SensePosition=on  SenseVelocity=on  SenseAcceleration=off  SenseTorqueForce=off  PositionTargetValue=MX28_init_position  PositionTargetValueUnits=rad  PositionTargetSpecify=on  PositionTargetPriority=High  VelocityTargetValue=MX28_init_speed  VelocityTargetValueUnits=rad/s  VelocityTargetSpecify=on  VelocityTargetPriority=High  BlockFunction=simmechanics.library.joints.revolute_joint
  Speed converter : nesl_utility/PS-Simulink Converter  PhysicalDomain=network_engine_domain  SubClassName=ps_output  LeftPortType=input  RightPortType=output  PseudoPeriodic=off  Frequencies=[]  Unit=rad/s  AffineConversion=off
  Torque converter : nesl_utility/Simulink-PS Converter  PhysicalDomain=network_engine_domain  SubClassName=ps_input  LeftPortType=input  RightPortType=output  PseudoPeriodic=off  Frequencies=[]  NoiseDistribution=none  NoiseParameters=[]  Unit=N*m  AffineConversion=off  InputFiltering=off  SimscapeFilterOrder=1  InputFilterTimeConstant=0.001  UdotUserProvided=1
  Base : PMIOPort  Port=1  Side=Left
  Axis : PMIOPort  Port=2  Side=Right
  wires:
  Model/4 -> MX28 State/3
  Model/2 -> MX28 State/1
  Model/5 -> MX28 State/4
  Model/3 -> MX28 State/2
  MX28 Command/3 -> Model/5
  MX28 Command/6 -> Model/8
  MX28 Command/4 -> Model/6
  MX28 Command/5 -> Model/7
  MX28 Command/7 -> Model/9
  MX28 Command/2 -> Model/4
  MX28 Command/1 -> Model/3
  Position converter/1 -> Model/2
  Speed converter/1 -> Model/1
  Model/1 -> Torque converter/1
  Model/6 -> MX28 State/5
  MX28 Command/8 -> Model/10
  MX28 Command/9 -> Model/11
  connections:
  Axis/RConn1 -- Revolute Joint/RConn1 -- Inertia/RConn1
  Revolute Joint/LConn1 -- Base/RConn1
  Revolute Joint/RConn3 -- Speed converter/LConn1
  Revolute Joint/RConn2 -- Position converter/LConn1
  Revolute Joint/LConn2 -- Torque converter/RConn1

== system left_leg/Left Leg/Left Hip Yaw ==
  Left Hip Yaw Axis to Left Hip Roll Axis : sm_lib/Frames and Transforms/Rigid Transform  TranslationMethod=Cartesian  TranslationLengthUnit=mm  TranslationStandardAxis=+Z  TranslationStandardOffset=0  TranslationCartesianOffset=[24.85 0 28.35]  TranslationROffset=0  TranslationROffsetUnits=m  TranslationZOffset=0  TranslationZOffsetUnits=m  TranslationThetaOffset=0  TranslationThetaOffsetUnits=deg  RotationMethod=AlignedAxes  RotationAngleUnits=deg  RotationStandardAxis=+Z  RotationAngle=0  RotationArbitraryAxis=[0 0 1]  FollAlignAxisA=+Y  BaseAlignAxisA=+Z  FollAlignAxisB=+X  BaseAlignAxisB=-Y  RotationMatrix=[1 0 0; 0 1 0; 0 0 1]  BlockFunction=simmechanics.library.frames_transforms.rigid_transform
  Solid : sm_lib/Body Elements/Solid  InertiaType=Custom  Mass=34.1  MassUnits=g  CenterOfMass=[7.53 0 10.27]  CenterOfMassUnits=mm  MomentsOfInertia=[8263 18980 13482]  MomentsOfInertiaUnits=g*mm^2  ProductsOfInertia=[0 3667 0]  ProductsOfInertiaUnits=g*mm^2  DensityBased=on  Density=1000  DensityUnits=kg/(m^3)  GraphicType=FromGeometry  MarkerShape=Sphere  MarkerSize=10  MarkerSizeUnits=m  GraphicVisPropType=SimpleVisualProperties  GraphicDiffuseColor=[0.5 0.5 0.5]  GraphicSpecularColor=[0.5 0.5 0.5 1.0]  GraphicAmbientColor=[0.15 0.15 0.15 1.0]  GraphicEmissiveColor=[0.0 0.0 0.0 1.0]  GraphicShininess=75  GraphicOpacity=1.0  GeometryShape=FromFile  RectangleSize=[1 1]  RectangleSizeUnits=m  BrickDimensions=[1 1 1]  BrickDimensionUnits=mm  CylinderRadius=1  CylinderRadiusUnits=m  CylinderLength=1  CylinderLengthUnits=m  SphereRadius=1  SphereRadiusUnits=m  EllipsoidRadii=[1 1 1]  EllipsoidRadiiUnits=m  ExtrusionCrossSection=[1 1; -1 1; -1 -1; 1 -1]  ExtrusionCrossSectionUnits=m  ExtrusionLength=1  ExtrusionLengthUnits=m  PolygonNumSides=3  PolygonOuterRadius=1  PolygonOuterRadiusUnits=m  ExtGeomFileType=STL  ExtGeomFileName=D:\Ker Lann\systemes\darwin\kinematics\STL\Hip1.STL  ExtGeomFileUnits=mm  RevolutionCrossSection=[1 1; 1 -1; 2 -1; 2 1]  RevolutionCrossSectionUnits=m  RevolutionExtent=Full  RevolutionAngle=180  RevolutionAngleUnits=deg  BlockFunction=simmechanics.library.body_elements.solid
  Left Hip Yaw : PMIOPort  Port=1  Side=Left
  Left Hip Roll : PMIOPort  Port=2  Side=Right
  connections:
  Left Hip Yaw/RConn1 -- Solid/RConn1 -- Left Hip Yaw Axis to Left Hip Roll Axis/LConn1
  Left Hip Yaw Axis to Left Hip Roll Axis/RConn1 -- Left Hip Roll/RConn1

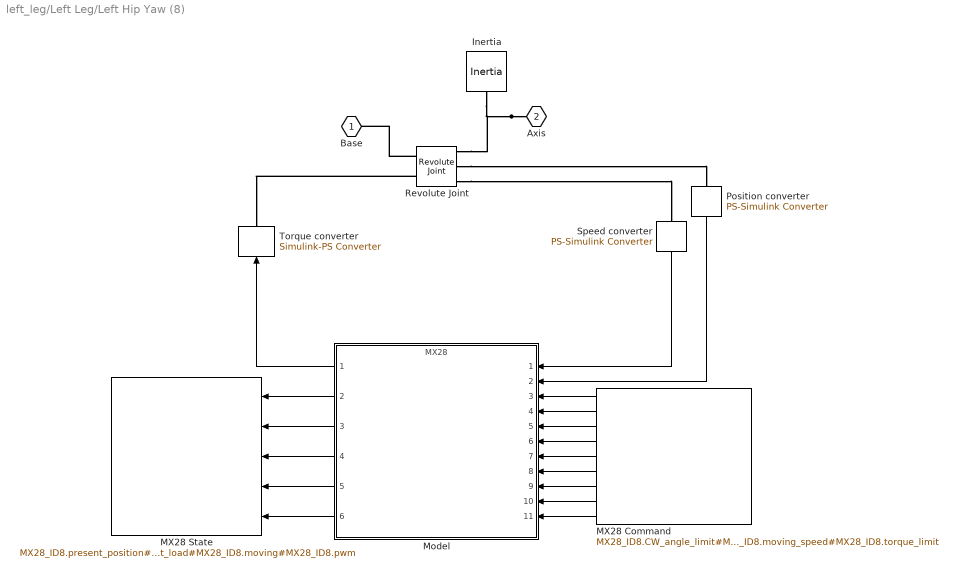
== system left_leg/Left Leg/Left Hip Yaw (8) ==
  Inertia : sm_lib/Body Elements/Inertia  InertiaType=Custom  Mass=1  MassUnits=g  CenterOfMass=[0 0 0]  CenterOfMassUnits=m  MomentsOfInertia=[0 0 MX28_inertia]  MomentsOfInertiaUnits=kg*m^2  ProductsOfInertia=[0 0 0]  ProductsOfInertiaUnits=kg*m^2  BlockFunction=simmechanics.library.body_elements.inertia
  MX28 Command : DataStoreRead  DataStoreName=MX28_ID8  SampleTime=MX28_Te  DataStoreElements=MX28_ID8.CW_angle_limit#MX28_ID8.CCW_angle_limit#MX28_ID8.torque_enable#MX28_ID8.D_gain#MX28_ID8.I_gain#MX28_ID8.P_gain#MX28_ID8.goal_position#MX28_ID8.moving_speed#MX28_ID8.torque_limit
  MX28 State : DataStoreWrite  DataStoreName=MX28_ID8  DataStoreElements=MX28_ID8.present_position#MX28_ID8.present_speed#MX28_ID8.present_load#MX28_ID8.moving#MX28_ID8.pwm
  Model : ModelReference  ModelNameDialog=MX28.slx  SimulationMode=Normal  ModelReferenceVersion=1.66  CopyOfModelName=MX28.slx  DefaultDataLogging=on
  Position converter : nesl_utility/PS-Simulink Converter  PhysicalDomain=network_engine_domain  SubClassName=ps_output  LeftPortType=input  RightPortType=output  PseudoPeriodic=off  Frequencies=[]  Unit=rad  AffineConversion=off
  Revolute Joint : sm_lib/Joints/Revolute Joint  SenseConstraintForce=off  SenseConstraintForceX=off  SenseConstraintForceY=off  SenseConstraintForceZ=off  SenseConstraintTorque=off  SenseConstraintTorqueX=off  SenseConstraintTorqueY=off  SenseConstraintTorqueZ=off  SenseTotalForce=off  SenseTotalForceX=off  SenseTotalForceY=off  SenseTotalForceZ=off  SenseTotalTorque=off  SenseTotalTorqueX=off  SenseTotalTorqueY=off  SenseTotalTorqueZ=off  CompositeWrenchDir=FollowerOnBase  CompositeWrenchFrame=BaseFrame  EquilibriumPosition=0  EquilibriumPositionUnits=deg  SpringStiffness=0  SpringStiffnessUnits=N*m/deg  DampingCoefficient=MX28_lub_friction  DampingCoefficientUnits=N*m/(rad/s)  TorqueActuationMode=InputTorque  MotionActuationMode=ComputedMotion  SensePosition=on  SenseVelocity=on  SenseAcceleration=off  SenseTorqueForce=off  PositionTargetValue=MX28_init_position  PositionTargetValueUnits=rad  PositionTargetSpecify=on  PositionTargetPriority=High  VelocityTargetValue=MX28_init_speed  VelocityTargetValueUnits=rad/s  VelocityTargetSpecify=on  VelocityTargetPriority=High  BlockFunction=simmechanics.library.joints.revolute_joint
  Speed converter : nesl_utility/PS-Simulink Converter  PhysicalDomain=network_engine_domain  SubClassName=ps_output  LeftPortType=input  RightPortType=output  PseudoPeriodic=off  Frequencies=[]  Unit=rad/s  AffineConversion=off
  Torque converter : nesl_utility/Simulink-PS Converter  PhysicalDomain=network_engine_domain  SubClassName=ps_input  LeftPortType=input  RightPortType=output  PseudoPeriodic=off  Frequencies=[]  NoiseDistribution=none  NoiseParameters=[]  Unit=N*m  AffineConversion=off  InputFiltering=off  SimscapeFilterOrder=1  InputFilterTimeConstant=0.001  UdotUserProvided=1
  Base : PMIOPort  Port=1  Side=Left
  Axis : PMIOPort  Port=2  Side=Right
  wires:
  Model/4 -> MX28 State/3
  Model/2 -> MX28 State/1
  Model/5 -> MX28 State/4
  Model/3 -> MX28 State/2
  MX28 Command/3 -> Model/5
  MX28 Command/6 -> Model/8
  MX28 Command/4 -> Model/6
  MX28 Command/5 -> Model/7
  MX28 Command/7 -> Model/9
  MX28 Command/2 -> Model/4
  MX28 Command/1 -> Model/3
  Speed converter/1 -> Model/1
  Position converter/1 -> Model/2
  Model/1 -> Torque converter/1
  Model/6 -> MX28 State/5
  MX28 Command/8 -> Model/10
  MX28 Command/9 -> Model/11
  connections:
  Axis/RConn1 -- Revolute Joint/RConn1 -- Inertia/RConn1
  Revolute Joint/LConn1 -- Base/RConn1
  Revolute Joint/RConn3 -- Speed converter/LConn1
  Revolute Joint/RConn2 -- Position converter/LConn1
  Revolute Joint/LConn2 -- Torque converter/RConn1
